simulink model "regionselector"  (R2012b)
settings: Solver=ode1  StartTime=0.0  StopTime=inf  FixedStep=0.002  RelTol=1e-3
settings Model: ExtModeTrigDuration=5000  Creator=Vicon  LastModifiedBy=Vicon
settings SolverCC: PositivePriorityOrder=on
settings RTWCC: SystemTargetFile=quarc_win64.tlc  TemplateMakefile=quarc_default_tmf  Description=QUARC Win64 Target  ProcessScript=quarc_win64_make_rtw_hook
settings STFCustomTargetCC: TargetPreCompLibLocation=C:\PROGRA~3\QUARC\lib\2012b\win64\release  CodeReplacementLibrary=ANSI_C  GeneratePreprocessorConditionals=Disable all  CombineOutputUpdateFcns=on  GRTInterface=off  SystemTargetFile=quarc_win64.tlc
settings GRTTargetCC: TargetPreCompLibLocation=C:\PROGRA~3\QUARC\lib\2012b\win64\release  ParMdlRefBuildCompliant=off  CompOptLevelCompliant=off  ConcurrentExecutionCompliant=off  MatFileLogging=off  ExtMode=on  ExtModeMexFile=quarc_comm

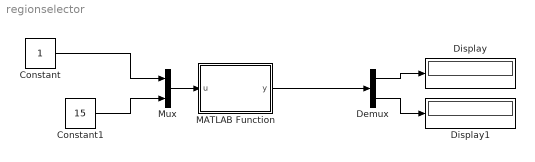
== system regionselector ==
  Constant : Constant
  Constant1 : Constant  Value=15
  Demux : Demux  Outputs=2
  Display : Display
  Display1 : Display
  MATLAB Function : MATLAB Function  TreatAsAtomicUnit=on
  Mux : Mux  Inputs=2
  wires:
  Mux/1 -> MATLAB Function/1(u)
  Constant/1 -> Mux/1
  Constant1/1 -> Mux/2
  MATLAB Function/1(y) -> Demux/1
  Demux/1 -> Display/1
  Demux/2 -> Display1/1

== matlab function regionselector/MATLAB Function ==
  data: u input; y output
function y = fcn(u)
%#codegen
